simulink model "MatlabFunctionexp1"  (R2015b)
settings: Solver=VariableStepAuto  StartTime=0.0  StopTime=10.0  RelTol=1e-3
settings Model: Creator=LUBO  LastModifiedBy=LUBO

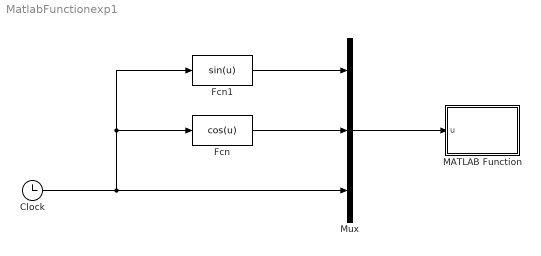
== system MatlabFunctionexp1 ==
  Clock : Clock
  Fcn : Fcn  Expr=cos(u)
  Fcn1 : Fcn  Expr=sin(u)
  MATLAB Function : MATLAB Function  TreatAsAtomicUnit=on
  Mux : Mux  Inputs=3
  wires:
  Clock/1 -> Fcn/1, Fcn1/1, Mux/3
  Fcn/1 -> Mux/2
  Fcn1/1 -> Mux/1
  Mux/1 -> MATLAB Function/1(u)

== matlab function MatlabFunctionexp1/MATLAB Function ==
  data: u input
function scope_3d(u)
%#codegen
eml.extrinsic('plot3','scatter3','close','delete');
len=length(u);
persistent data
if isempty(data)
    data=zeros(3,100000);%初始化一个足够大的的存储空间
end
persistent n             % count the input sample number
 if isempty(n)
     n=1;
 else
     n=n+1;
 end
 data(:,n)=u;

 persistent h 

 if isempty(h)
     h=plot3(data(1,:),data(2,:),data(3,:),'o'); 
     grid on
 else
     delete h;              %每个采样时刻都重新绘制图像已达到动态刷新的效果
     h=plot3(data(1,:),data(2,:),data(3,:),'o');
     grid on
 end
